simulink model "rc_node"  (Simulink 7.8)
settings: Solver=FixedStepDiscrete  SolverMode=SingleTasking  StartTime=0.0  StopTime=10.0  FixedStep=0.01  RelTol=1e-3
InitFcn:
  | clear all;
  | RcNodeInit
values from neighbouring files (symbols this model uses):
  MaxPwmIn = 0.0025    [RcNodeInit.m]
  T_step = 0.01    [RcNodeInit.m]
undefined symbols (not defined in the file or in its folder): Acs300SendThrottleCommand, ANmax, DataEEInitAndClear, DataStoreSaveParameters, DiscIntNeverNeededParam, Ecan1Init, IC1max, IC2max, IC7max, IC8max, Init_onlyOnce, Init_Reset, NodeTransmitStatus, RcNodeInit, RudderSendAngleCommand, RudderStartCalibration, TransmitStatus, u1, u2
libraries: simulink x35, dsPICdrivers x19, simulink_need_slupdate x1, ecan_dspic x1
(part 1 of 2)
CloseFcn:
  | rtwprivate ssgencode ModelCloseRequest rc_node
settings Model: Creator=bwmairs  LastModifiedBy=Bryant
settings OptimizationCC: BlockReduction=off  InlineParams=on  InlineInvariantSignals=on  PassReuseOutputArgsAs=Individual arguments  ZeroExternalMemoryAtStartup=off  ZeroInternalMemoryAtStartup=off  InitFltsAndDblsToZero=on  NoFixptDivByZeroProtection=on  EfficientFloat2IntCast=on  OptimizeModelRefInitCode=on
settings DebuggingCC: ReadBeforeWriteMsg=DisableAll  WriteAfterWriteMsg=DisableAll  WriteAfterReadMsg=DisableAll  UnderspecifiedInitializationDetection=Simplified  ParameterOverflowMsg=warning  FcnCallInpInsideContextMsg=Use local settings  UniqueDataStoreMsg=error
settings HardwareCC: ProdBitPerInt=16  ProdBitPerPointer=16  ProdIntDivRoundTo=Zero  ProdEndianess=LittleEndian  ProdWordSize=16  ProdHWDeviceType=16-bit Generic
settings ModelReferenceCC: ModelReferenceNumInstancesAllowed=Single
settings SFSimCC: SimParseCustomCode=off
settings RTWCC: SystemTargetFile=dspic.tlc  GenCodeOnly=on  MakeCommand=make_CreateMPLAB  TemplateMakefile=dspic_pic30_gcc.tmf  PostCodeGenCommand=dsPIC_Compile()  Description=Embedded Target for Microchip dsPIC (real-time)  ProcessScript=dspic_make_rtw_hook  CustomInclude=../Libs/C  RTWCompilerOptimization=On
settings RTWCC: CustomSource=|
  | ../Libs/C/Conversions.c
  | ../Libs/C/Nmea2000.c
  | ../Libs/C/Nmea2000Encode.c
  | ../Libs/C/Uart1.c
  | ../Libs/C/DEE.c
  | ../Libs/C/DEES.s
  | ../Libs/C/Traps.c
  | ../Libs/C/CanMessages.c
  | ../Libs/C/Acs300.c
  | ../Libs/C/Rudder.c
  | ../Libs/C/Node.c
  | ../Libs/C/CircularBuffer.c
  | ../Libs/C/Ecan1.c
  | ../Libs/C/Parameters.c
  | ../Libs/C/DataStore.c
  | 
  | clib/RcNode.c
  | clib/ParametersHelper.c
settings CodeAppCC: IgnoreCustomStorageClasses=off  IgnoreTestpoints=on
settings STFCustomTargetCC: TargetFunctionLibrary=C89/C90 (ANSI)  IncludeMdlTerminateFcn=off  GeneratePreprocessorConditionals=Use local settings  CombineOutputUpdateFcns=on  SuppressErrorStatus=on  ERTCustomFileBanners=on  SupportComplex=off  SupportContinuousTime=off  SupportNonInlinedSFcns=off  SystemTargetFile=dspic.tlc
settings ERTTargetCC: TargetFunctionLibrary=C89/C90 (ANSI)  MultiwordLength=2048  ParMdlRefBuildCompliant=off  CompOptLevelCompliant=off  ConcurrentExecutionCompliant=off  IncludeMdlTerminateFcn=off  SuppressErrorStatus=on  ERTFirstTimeCompliant=off  SupportComplex=off  ModelStepFunctionPrototypeControlCompliant=off  CPPClassGenCompliant=off  ExtModeMexFile=ext_serial_win32_comm  InlinedParameterPlacement=NonHierarchical  ERTSrcFileBannerTemplate=dsPIC_code_template.cgt  ERTHdrFileBannerTemplate=dsPIC_code_template.cgt  ERTDataSrcFileTemplate=dsPIC_code_template.cgt  ERTDataHdrFileTemplate=dsPIC_code_template.cgt  ERTCustomFileTemplate=dsPIC_main.tlc  SuppressUnreachableDefaultCases=off
settings CustomProperty: DataType=string  Value=C:\PROGRA~1\MATLAB\R2011b\bin\win64\gmake

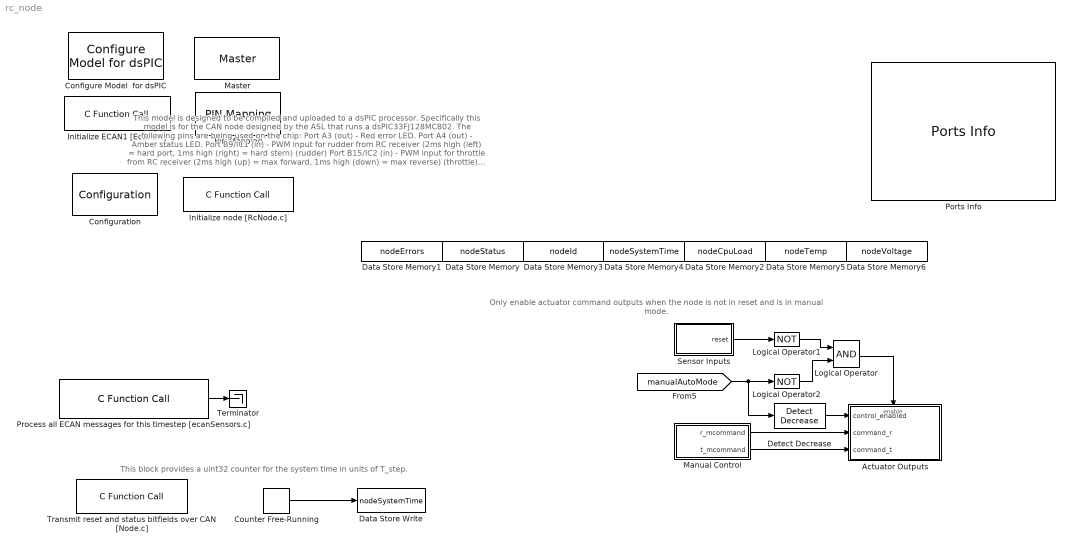
== system rc_node ==
  note: This model is designed to be compiled and uploaded to a dsPIC processor.
      | Specifically this model is for the CAN node designed by the ASL that runs a dsPIC33FJ128MC802.
      | The following pins are being used on the chip:
      | Port A3 (out) - Red error LED.
      | Port A4 (out) - Amber status LED.
      | Port B9/IC1 (in) - PWM input for rudder from RC receiver (2ms high (left) = hard port, 1ms high (right) = hard stern) (rudder)
      | Port B15/IC2 (in) - PWM input for throttle from RC receiver (2ms high (up) = max forward, 1ms high (down) = max reverse) (throttle)
      | Port B10/IC7 (in) - PWM input for control mode from RC receiver (2ms high (down) = manual control, 1ms high (up) = auto. control) (gear)
      | Ports B6/B7 (in/out) - Pins required for the ECAN1 peripheral. This is used for controlling the propeller motor.
      | Port B4/B5 (in/out) - UART1 transmission line.
      |
      | Switching between the autonomous controller and manual control involves using the landing gear channel. When
      | it's enabled, it's under autonomous control. This can only be changed when the RC transmitter is on and connected and
      | is never changed otherwise.
      |
      | Additionally a rudder calibration command can be sent by being in manual mode and toggling channel 5, the aileron channel, left-right-left.
      | To do it a second time you need to switch out of and back into manual mode.
  note: This block provides a uint32 counter for the system time in units of T_step.
  note: Only enable actuator command outputs when the node is not in
      | reset and is in manual mode.
  Actuator Outputs : Subsystem
  Configuration : dsPICdrivers/Configuration  double64=on
  Configure Model  for dsPIC : dsPICdrivers/Simulink Configuration/Configure Model  for dsPIC
  Counter Free-Running : simulink/Sources/Counter Free-Running  NumBits=32  tsamp=T_step
  Data Store Memory : DataStoreMemory  DataStoreName=nodeStatus  ReadBeforeWriteMsg=warning  WriteAfterWriteMsg=warning  WriteAfterReadMsg=warning  OutDataTypeStr=uint16
      settings: RTWStateStorageClass=ImportedExtern
  Data Store Memory1 : DataStoreMemory  DataStoreName=nodeErrors  ReadBeforeWriteMsg=warning  WriteAfterWriteMsg=warning  WriteAfterReadMsg=warning  OutDataTypeStr=uint16
      settings: RTWStateStorageClass=ImportedExtern
  Data Store Memory2 : DataStoreMemory  DataStoreName=nodeCpuLoad  ReadBeforeWriteMsg=warning  WriteAfterWriteMsg=warning  WriteAfterReadMsg=warning  OutDataTypeStr=uint8
      settings: RTWStateStorageClass=ImportedExtern
  Data Store Memory3 : DataStoreMemory  DataStoreName=nodeId  ReadBeforeWriteMsg=warning  WriteAfterWriteMsg=warning  WriteAfterReadMsg=warning  OutDataTypeStr=uint8
      settings: RTWStateStorageClass=ImportedExtern
  Data Store Memory4 : DataStoreMemory  DataStoreName=nodeSystemTime  ReadBeforeWriteMsg=warning  WriteAfterWriteMsg=warning  WriteAfterReadMsg=warning  OutDataTypeStr=uint32
      settings: RTWStateStorageClass=ImportedExtern
  Data Store Memory5 : DataStoreMemory  DataStoreName=nodeTemp  ReadBeforeWriteMsg=warning  WriteAfterWriteMsg=warning  WriteAfterReadMsg=warning  OutDataTypeStr=int8
      settings: RTWStateStorageClass=ImportedExtern
  Data Store Memory6 : DataStoreMemory  DataStoreName=nodeVoltage  ReadBeforeWriteMsg=warning  WriteAfterWriteMsg=warning  WriteAfterReadMsg=warning  OutDataTypeStr=uint8
      settings: RTWStateStorageClass=ImportedExtern
  Data Store Write : DataStoreWrite  DataStoreName=nodeSystemTime
  Detect Decrease : simulink/Logic and Bit Operations/Detect Decrease  vinit=0.0  InputProcessing=Inherited  OutDataTypeStr=uint8
  Initialize ECAN1 [Ecan1.c] : dsPICdrivers/OTHERS/C Function Call  Tag=dsPIC_dsPIC_CFunctionCall  FctUpdate=None  fctName=Ecan1Init  INPUT_SIZE=1  INPUT1=--  INPUT2=--  INPUT3=--  OUTPUT_SIZE=1  OUTPUT1=--  SampleTime=Inf  InputType=[]  OutputType=[]  FctDeclaration=extern void Ecan1Init();  FctCall=Ecan1Init();  OrderingInOutPopup=None  FctStart=Start Function (Call once and only once)  FctStart_Name=Ecan1Init  FctStart_Declaration=inline extern void Ecan1Init();  FctStart_Call=Ecan1Init();  FctInit=None  FctInit_Name=Init_Reset  FctInit_Declaration=inline extern void Init_Reset();  FctInit_Call=Init_Reset();  PinDigitalInput=[]  PinDigitalOutput=[]  AnalogueInput=[]
  Initialize node [RcNode.c] : dsPICdrivers/OTHERS/C Function Call  Tag=dsPIC_dsPIC_CFunctionCall  FctUpdate=None  fctName=TransmitStatus  INPUT_SIZE=1  INPUT1=--  INPUT2=--  INPUT3=--  OUTPUT_SIZE=1  OUTPUT1=--  SampleTime=-1  InputType=[]  OutputType=[]  FctDeclaration=extern void TransmitStatus();  FctCall=TransmitStatus();  OrderingInOutPopup=None  FctStart=Start Function (Call once and only once)  FctStart_Name=RcNodeInit  FctStart_Declaration=inline extern void RcNodeInit();  FctStart_Call=RcNodeInit();  FctInit=None  FctInit_Name=Init_Reset  FctInit_Declaration=inline extern void Init_Reset();  FctInit_Call=Init_Reset();  PinDigitalInput=[]  PinDigitalOutput=[]  AnalogueInput=[]
  Logical Operator : Logic  AllPortsSameDT=off  OutDataTypeStr=boolean
  Logical Operator1 : Logic  Operator=NOT  AllPortsSameDT=off  OutDataTypeStr=boolean
  Logical Operator2 : Logic  Operator=NOT  AllPortsSameDT=off  OutDataTypeStr=boolean
  Manual Control : Subsystem
  Master : dsPICdrivers/Master  Tag=dsPIC_MASTER  Priority=1  TimeStepType=Timer1  picType=33fj128MC802  fcy=40008571.4286  Quartz_33f=8e6  PLLActive_33f=on  fcyDesired_33f=40000000  tmr1="[8  50010  -0.00057131]"  tmr1Info="Time Step : 0.01  ;   Error : -0.00057131%  PR1=50010"  tmr2345="[8  0  0  0]"  tmr2345cfg=[-1 -1 -1 -1]  IOautoConf=on  typePort="[ 0   8   0  10  10   0   0   0   0   0   0   0   0   0   0   0   0   0   0   8  22   0   0  23   0  22  22   0   0   0  22  22   0   0   0   0   0   0   0   0   0   0   0   0   0   0   0   0   0   0   0   0   0   0   0   0   0   0   0   0   0   0   0   0   0   0   0   0   0   0   0   0   0   0   0   0   0   0   0   0   0   0   0   0   0   0   0   0   0   0   0   0   0   0   0   0   0   0   0   0   0   0   0   0   0   0   0   0   0   0   0   0 ]"  TRIS="[ 65511  65407  65535  65535  65535  65535  65535 ]"  ADPCFG=0  MasterBusyPort=None  MasterOverloadPort=None  FOSC=Internal Fast RC 7.37Mhz  ClockSwitchMonitor=Both disabled  TempProtection_33f=TEMP_ON  FPBOR=<empty>  PWRT=disable  MCLR=<empty>  ICD=ICS_PGD3  JTAGEN=JTAGEN_OFF  PowerSave=off  OverrideFcy=off  NewFcy=1e6  PR2345="[65535  65535  65535  65535]"
  PIN Mapping : dsPICdrivers/Peripheral MAPPING/PIN Mapping  Tag=dsPIC_PIN_Mapping  in_INT1=Not tied (VSS)  in_INT2=Not tied (VSS)  in_T2CK=Not tied (VSS)  in_T3CK=Not tied (VSS)  in_T4CK=Not tied (VSS)  in_T5CK=Not tied (VSS)  in_IC1=tied to RP9  in_IC2=tied to RP15  in_IC7=tied to RP10  in_IC8=tied to RP14  out_OC1=Not changed  out_OC2=Not changed  out_OC3=Not changed  out_OC4=Not changed  in_OCFA=Not tied (VSS)  in_FLTA1=Not tied (VSS)  in_FLTA2=Not tied (VSS)  in_QEA1=Not tied (VSS)  in_QEB1=Not tied (VSS)  in_INDX1=Not tied (VSS)  out_UPDN1=Not changed  out_UPDN2=Not changed  in_QEA2=Not tied (VSS)  in_QEB2=Not tied (VSS)  in_INDX2=Not tied (VSS)  in_U1RX=Not changed  out_U1TX=Not changed  in_U1CTS=Not tied (VSS)  out_U1RTS=Not changed  in_U2RX=Not changed  out_U2TX=Not changed  in_U2CTS=Not tied (VSS)  out_U2RTS=Not changed  in_SDI1=Not tied (VSS)  out_SDO1=Not changed  in_SCK1=Not tied (VSS)  out_SCK1OUT=Not changed  in_SS1=Not tied (VSS)  out_SS1OUT=Not changed  in_SDI2=Not tied (VSS)  out_SDO2=Not changed  in_SCK2=Not tied (VSS)  out_SCK2OUT=Not changed  in_SS2=Not tied (VSS)  out_SS2OUT=Not changed  in_C1RX=tied to RP4  out_C1TX=tied to RP7  out_C1OUT=Not changed  out_C2OUT=Not changed
  Ports Info : dsPICdrivers/Ports Info  Tag=dsPIC_PortInfo
  Process all ECAN messages for this timestep [ecanSensors.c] : dsPICdrivers/OTHERS/C Function Call  Tag=dsPIC_dsPIC_CFunctionCall  FctUpdate=Output Function  fctName=ProcessAllEcanMessages  INPUT_SIZE=1  INPUT1=--  INPUT2=--  INPUT3=--  OUTPUT_SIZE=1  OUTPUT1=uint8  SampleTime=T_step  InputType=[ ]  OutputType=[ 2 ]  FctDeclaration=extern uint8_T ProcessAllEcanMessages();  FctCall=%y1 = ProcessAllEcanMessages();  OrderingInOutPopup=None  FctStart=None  FctStart_Name=Init_onlyOnce  FctStart_Declaration=inline extern void Init_onlyOnce();  FctStart_Call=Init_onlyOnce();  FctInit=None  FctInit_Name=Init_Reset  FctInit_Declaration=inline extern void Init_Reset();  FctInit_Call=Init_Reset();  PinDigitalInput=[]  PinDigitalOutput=[]  AnalogueInput=[]
  Sensor Inputs : Subsystem
  Terminator : Terminator
  Transmit reset and status bitfields over CAN [Node.c] : dsPICdrivers/OTHERS/C Function Call  Tag=dsPIC_dsPIC_CFunctionCall  FctUpdate=Output Function  fctName=NodeTransmitStatus  INPUT_SIZE=1  INPUT1=--  INPUT2=--  INPUT3=--  OUTPUT_SIZE=1  OUTPUT1=--  SampleTime=0.5  InputType=[ ]  OutputType=[ ]  FctDeclaration=extern void NodeTransmitStatus();  FctCall=NodeTransmitStatus();  OrderingInOutPopup=None  FctStart=None  FctStart_Name=DataEEInitAndClear  FctStart_Declaration=inline extern void DataEEInitAndClear();  FctStart_Call=DataEEInitAndClear();  FctInit=None  FctInit_Name=Init_Reset  FctInit_Declaration=inline extern void Init_Reset();  FctInit_Call=Init_Reset();  PinDigitalInput=[]  PinDigitalOutput=[]  AnalogueInput=[]
  wires:
  Process all ECAN messages for this timestep [ecanSensors.c]/1 -> Terminator/1
  Sensor Inputs/1(reset) -> Logical Operator1/1
  Manual Control/1(r_mcommand) -> Actuator Outputs/2(command_r)
  Manual Control/2(t_mcommand) -> Actuator Outputs/3(command_t)
  Logical Operator1/1 -> Logical Operator/1
  Counter Free-Running/1 -> Data Store Write/1
  [manualAutoMode] -> Logical Operator2/1, Detect Decrease/1
  Logical Operator/1 -> Actuator Outputs/Enable
  Logical Operator2/1 -> Logical Operator/2
  Detect Decrease/1 -> Actuator Outputs/1(control_enabled)

== system rc_node/Actuator Outputs ==
  note: Propulsion is controlled here via a CAN interface to the motor driver board.
      | ECAN1 is used and several possible commands are transmitted: enable, disable,
      | or change speed, with speed being between -1023 and 1023 taken as a fraction
      | of total speed (1023).
  note: Rudder commands are controlled via a CAN interface to a CAN_node controller
      | at the stern of the vessel.
  note: Actuator messages are only transmit when the command signal has changed,
      | though when the device is switched over to manual control, messages are
      | transmit as well.
  control_enabled : Inport
  command_r : Inport  Port=2
  command_t : Inport  Port=3
  Enable : EnablePort
  Detect Change : simulink/Logic and Bit Operations/Detect Change  vinit=0  InputProcessing=Inherited  OutDataTypeStr=uint8
  Detect Change1 : simulink/Logic and Bit Operations/Detect Change  vinit=0  InputProcessing=Inherited  OutDataTypeStr=uint8
  Logical Operator : Logic  Operator=OR  AllPortsSameDT=off  OutDataTypeStr=boolean
  Logical Operator1 : Logic  Operator=OR  AllPortsSameDT=off  OutDataTypeStr=boolean
  Transmit Angle Command : Subsystem  TreatAsAtomicUnit=on
  Transmit Throttle Command : Subsystem  TreatAsAtomicUnit=on
  wires:
  command_r/1 -> Detect Change/1, Transmit Angle Command/1(r_angle)
  command_t/1 -> Transmit Throttle Command/1(t_cmd), Detect Change1/1
  Logical Operator/1 -> Transmit Angle Command/Trigger
  Detect Change/1 -> Logical Operator/2
  control_enabled/1 -> Logical Operator/1, Logical Operator1/1
  Logical Operator1/1 -> Transmit Throttle Command/Trigger
  Detect Change1/1 -> Logical Operator1/2

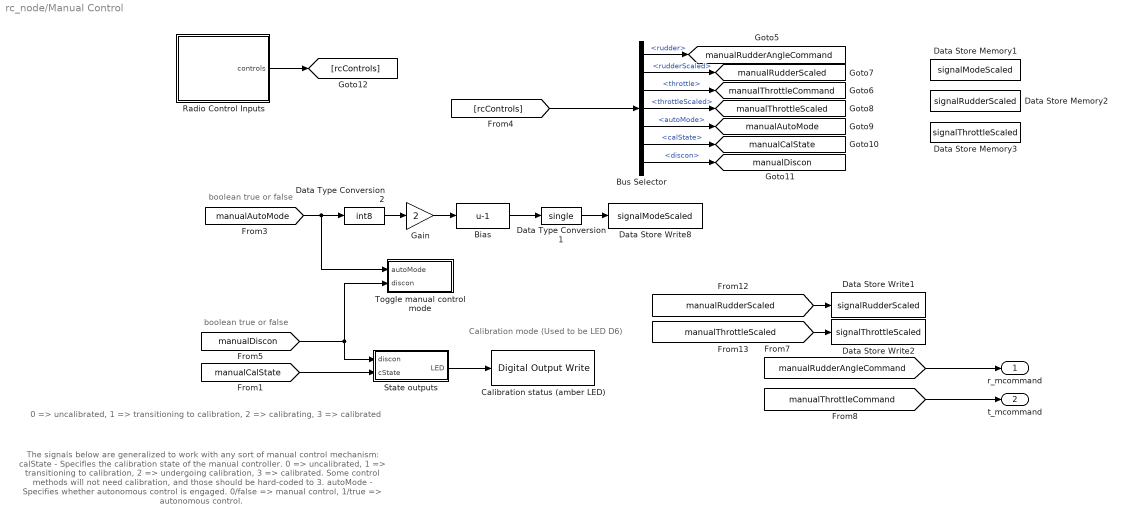
== system rc_node/Manual Control ==
  note: The signals below are generalized to work with any sort of manual control mechanism:
      | calState - Specifies the calibration state of the manual controller.
      |                 0 => uncalibrated, 1 => transitioning to calibration, 2 => undergoing calibration, 3 => calibrated. Some control methods will not need calibration, and those should be hard-coded to 3.
      | autoMode - Specifies whether autonomous control is engaged. 0/false => manual control, 1/true => autonomous control.
  note: boolean true or false
  note: boolean true or false
  note: 0 => uncalibrated,
      | 1 => transitioning to calibration,
      | 2 => calibrating,
      | 3 => calibrated
  note: Calibration mode
      | (Used to be LED D6)
  Bias : Bias  Bias=-1
  Bus Selector : BusSelector  OutputSignals=rudder,rudderScaled,throttle,throttleScaled,autoMode,calState,discon
  Calibration status (amber LED) : dsPICdrivers/Digital I//O/Digital Output Write  Tag=dsPIC_Digital_Output  Priority=5  PORT=A  Pin=[4]  Simultaneous=off  OrderingInOutPopup=None
  Data Store Memory1 : DataStoreMemory  DataStoreName=signalModeScaled  ReadBeforeWriteMsg=warning  WriteAfterWriteMsg=warning  WriteAfterReadMsg=warning  OutDataTypeStr=single
      settings: RTWStateStorageClass=ExportedGlobal
  Data Store Memory2 : DataStoreMemory  DataStoreName=signalRudderScaled  ReadBeforeWriteMsg=warning  WriteAfterWriteMsg=warning  WriteAfterReadMsg=warning  OutDataTypeStr=single
      settings: RTWStateStorageClass=ExportedGlobal
  Data Store Memory3 : DataStoreMemory  DataStoreName=signalThrottleScaled  ReadBeforeWriteMsg=warning  WriteAfterWriteMsg=warning  WriteAfterReadMsg=warning  OutDataTypeStr=single
      settings: RTWStateStorageClass=ExportedGlobal
  Data Store Write1 : DataStoreWrite  DataStoreName=signalRudderScaled
  Data Store Write2 : DataStoreWrite  DataStoreName=signalThrottleScaled
  Data Store Write8 : DataStoreWrite  DataStoreName=signalModeScaled  DataStoreElements=signalModeScaled
  Data Type Conversion1 : DataTypeConversion  OutDataTypeStr=single  RndMeth=Simplest
  Data Type Conversion2 : DataTypeConversion  OutDataTypeStr=int8  RndMeth=Simplest
  Gain : Gain  Gain=2  OutDataTypeStr=Inherit: Same as input  ParamDataTypeStr=Inherit: Same as input
  Radio Control Inputs : Subsystem
  State outputs : Subsystem
  Toggle manual control mode : Subsystem
  r_mcommand : Outport
  t_mcommand : Outport  Port=2
  tag scope: manualAutoMode=global, manualCalState=global, manualDiscon=global, manualRudderAngleCommand=global, manualRudderScaled=global, manualThrottleCommand=global, manualThrottleScaled=global
  wires:
  State outputs/1(LED) -> Calibration status (amber LED)/1
  Bias/1 -> Data Type Conversion1/1
  Gain/1 -> Bias/1
  Radio Control Inputs/1(controls) -> [rcControls]
  Bus Selector/1 -> [manualRudderAngleCommand]  "<rudder>"
  Bus Selector/3 -> [manualThrottleCommand]  "<throttle>"
  Bus Selector/2 -> [manualRudderScaled]  "<rudderScaled>"
  Bus Selector/4 -> [manualThrottleScaled]  "<throttleScaled>"
  Bus Selector/5 -> [manualAutoMode]  "<autoMode>"
  Bus Selector/6 -> [manualCalState]  "<calState>"
  Bus Selector/7 -> [manualDiscon]  "<discon>"
  [manualAutoMode] -> Data Type Conversion2/1, Toggle manual control mode/1(autoMode)
  [manualDiscon] -> State outputs/1(discon), Toggle manual control mode/2(discon)
  [manualCalState] -> State outputs/2(cState)
  [manualRudderAngleCommand] -> r_mcommand/1
  [manualThrottleCommand] -> t_mcommand/1
  [manualThrottleScaled] -> Data Store Write2/1
  [manualRudderScaled] -> Data Store Write1/1
  [rcControls] -> Bus Selector/1
  Data Type Conversion1/1 -> Data Store Write8/1
  Data Type Conversion2/1 -> Gain/1

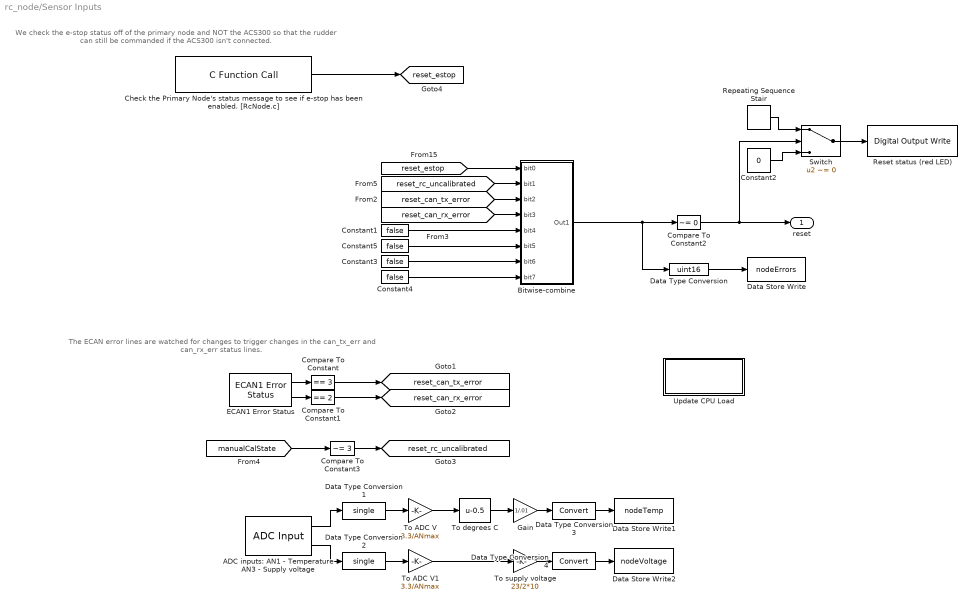
== system rc_node/Sensor Inputs ==
  note: The ECAN error lines are watched for changes to trigger changes
      | in the can_tx_err and can_rx_err status lines.
  note: We check the e-stop status off of the primary node and NOT the ACS300 so that
      | the rudder can still be commanded if the ACS300 isn't connected.
  ADC inputs: AN1 - Temperature AN3 - Supply voltage : dsPICdrivers/Peripheral I//O/ADC Input  Tag=dsPIC_ADC  Priority=5  ADC_TYPE=12 bits  ADC_MODE=Continuous sampling & get last channel value  NbrSampleStep=1  VoltRefpopup="AVdd  -  AVss"  OutFormatBitspopup=0000 dddd dddd dddd : Integer  InterruptPriority=6  ANCHANNELS=[1 5]  MaxName=ANmax = 4095  Rin=0  ADCS=53  SAMC=1  Temperature=25  DMAChannel=7  SampleTime=T_step  Status="OK  |  Tsmp=6.749e-007 |  T/Channel=1.012e-005 |  Tall=2.025e-005"  SSRC=auto convert
  Bitwise-combine : Subsystem
  Check the Primary Node's status message to see if e-stop has been enabled. [RcNode.c] : dsPICdrivers/OTHERS/C Function Call  Tag=dsPIC_dsPIC_CFunctionCall  FctUpdate=Output Function  fctName=GetEstopStatus  INPUT_SIZE=1  INPUT1=--  INPUT2=--  INPUT3=--  OUTPUT_SIZE=1  OUTPUT1=uint8  SampleTime=T_step  InputType=[ ]  OutputType=[ 2 ]  FctDeclaration=extern uint8_T GetEstopStatus();  FctCall=%y1 = GetEstopStatus();  OrderingInOutPopup=None  FctStart=None  FctStart_Name=Init_onlyOnce  FctStart_Declaration=inline extern void Init_onlyOnce();  FctStart_Call=Init_onlyOnce();  FctInit=None  FctInit_Name=Init_Reset  FctInit_Declaration=inline extern void Init_Reset();  FctInit_Call=Init_Reset();  PinDigitalInput=[]  PinDigitalOutput=[]  AnalogueInput=[]
  Compare To Constant : simulink/Logic and Bit Operations/Compare To Constant  relop===  const=3  OutDataTypeStr=boolean
  Compare To Constant1 : simulink/Logic and Bit Operations/Compare To Constant  relop===  const=2  OutDataTypeStr=boolean
  Compare To Constant2 : simulink/Logic and Bit Operations/Compare To Constant  relop=~=  const=0  OutDataTypeStr=boolean
  Compare To Constant3 : simulink/Logic and Bit Operations/Compare To Constant  relop=~=  const=3  OutDataTypeStr=boolean
  Constant{1,3..5} (4 alike) : Constant  Value=false  OutDataTypeStr=boolean
  Constant2 : Constant  Value=0  OutDataTypeStr=boolean
  Data Store Write : DataStoreWrite  DataStoreName=nodeErrors
  Data Store Write1 : DataStoreWrite  DataStoreName=nodeTemp
  Data Store Write2 : DataStoreWrite  DataStoreName=nodeVoltage
  Data Type Conversion : DataTypeConversion  OutDataTypeStr=uint16  RndMeth=Simplest
  Data Type Conversion1 : DataTypeConversion  OutDataTypeStr=single
  Data Type Conversion2 : DataTypeConversion  OutDataTypeStr=single
  Data Type Conversion3 : DataTypeConversion  RndMeth=Simplest
  Data Type Conversion4 : DataTypeConversion  RndMeth=Simplest
  ECAN1 Error Status : ecan_dspic/ECAN1 Error Status  ecan1_error_sample_time=T_step
  Gain : Gain  Gain=1/.01  RndMeth=Simplest
  Repeating Sequence Stair : simulink/Sources/Repeating Sequence Stair  OutValues=[1 0]  tsamp=.5  OutMin=[]  OutMax=[]  OutDataTypeStr=fixdt('boolean')  OutputDataTypeScalingMode=Specify via dialog  OutDataType=fixdt('boolean')  ConRadixGroup=Best Precision: Vector-wise  OutScaling=[]
  Reset status (red LED) : dsPICdrivers/Digital I//O/Digital Output Write  Tag=dsPIC_Digital_Output  Priority=5  PORT=A  Pin=[3]  Simultaneous=off  OrderingInOutPopup=None
  Switch : Switch  Criteria=u2 ~= 0
  To ADC V : Gain  Gain=3.3/ANmax
  To ADC V1 : Gain  Gain=3.3/ANmax
  To degrees C : Bias  Bias=-0.5
  To supply voltage : Gain  Gain=23/2*10  RndMeth=Simplest
  Update CPU Load : Subsystem
      mask Display: disp('');
  reset : Outport
  tag scope: reset_can_rx_error=global, reset_can_tx_error=global, reset_estop=global, reset_rc_uncalibrated=global
  wires:
  Check the Primary Node's status message to see if e-stop has been enabled. [RcNode.c]/1 -> [reset_estop]
  ECAN1 Error Status/1 -> Compare To Constant/1
  ECAN1 Error Status/2 -> Compare To Constant1/1
  Compare To Constant1/1 -> [reset_can_rx_error]
  Compare To Constant/1 -> [reset_can_tx_error]
  Constant2/1 -> Switch/3
  Repeating Sequence Stair/1 -> Switch/1
  Switch/1 -> Reset status (red LED)/1
  [reset_estop] -> Bitwise-combine/1(bit0)
  [reset_rc_uncalibrated] -> Bitwise-combine/2(bit1)
  [reset_can_tx_error] -> Bitwise-combine/3(bit2)
  [reset_can_rx_error] -> Bitwise-combine/4(bit3)
  Bitwise-combine/1(Out1) -> Compare To Constant2/1, Data Type Conversion/1
  Compare To Constant2/1 -> Switch/2, reset/1
  Constant3/1 -> Bitwise-combine/7(bit6)
  Constant4/1 -> Bitwise-combine/8(bit7)
  Data Type Conversion/1 -> Data Store Write/1
  Compare To Constant3/1 -> [reset_rc_uncalibrated]
  [manualCalState] -> Compare To Constant3/1
  Constant1/1 -> Bitwise-combine/5(bit4)
  Constant5/1 -> Bitwise-combine/6(bit5)
  To ADC V/1 -> To degrees C/1
  Data Type Conversion1/1 -> To ADC V/1
  ADC inputs: AN1 - Temperature AN3 - Supply voltage/1 -> Data Type Conversion1/1
  To degrees C/1 -> Gain/1
  Gain/1 -> Data Type Conversion3/1
  To ADC V1/1 -> To supply voltage/1
  Data Type Conversion2/1 -> To ADC V1/1
  To supply voltage/1 -> Data Type Conversion4/1
  ADC inputs: AN1 - Temperature AN3 - Supply voltage/2 -> Data Type Conversion2/1
  Data Type Conversion3/1 -> Data Store Write1/1
  Data Type Conversion4/1 -> Data Store Write2/1

== system rc_node/Actuator Outputs/Transmit Angle Command ==
  r_angle : Inport
  Trigger : TriggerPort
  Data Store Read1 : DataStoreRead  DataStoreName=nodeId
  Transmit rudder angle command [Rudder.c] : dsPICdrivers/OTHERS/C Function Call  Tag=dsPIC_dsPIC_CFunctionCall  FctUpdate=Output Function  fctName=RudderSendAngleCommand  INPUT_SIZE=1  INPUT1=uint8  INPUT2=real32  INPUT3=--  OUTPUT_SIZE=1  OUTPUT1=--  SampleTime=-1  InputType=[ 2 7 ]  OutputType=[ ]  FctDeclaration=extern void RudderSendAngleCommand(uint8_T u1, real32_T u2);  FctCall=RudderSendAngleCommand(%u1, %u2);  OrderingInOutPopup=None  FctStart=None  FctStart_Name=Init_onlyOnce  FctStart_Declaration=inline extern void Init_onlyOnce();  FctStart_Call=Init_onlyOnce();  FctInit=None  FctInit_Name=Init_Reset  FctInit_Declaration=inline extern void Init_Reset();  FctInit_Call=Init_Reset();  PinDigitalInput=[]  PinDigitalOutput=[]  AnalogueInput=[]
  wires:
  r_angle/1 -> Transmit rudder angle command [Rudder.c]/2
  Data Store Read1/1 -> Transmit rudder angle command [Rudder.c]/1

== system rc_node/Actuator Outputs/Transmit Throttle Command ==
  t_cmd : Inport
  Trigger : TriggerPort
  Transmit throttle angle command [Acs300.c] : dsPICdrivers/OTHERS/C Function Call  Tag=dsPIC_dsPIC_CFunctionCall  FctUpdate=Output Function  fctName=Acs300SendThrottleCommand  INPUT_SIZE=1  INPUT1=int16  INPUT2=--  INPUT3=--  OUTPUT_SIZE=1  OUTPUT1=--  SampleTime=-1  InputType=[ 3 ]  OutputType=[ ]  FctDeclaration=extern void Acs300SendThrottleCommand(int16_T u1);  FctCall=Acs300SendThrottleCommand(%u1);  OrderingInOutPopup=None  FctStart=None  FctStart_Name=Init_onlyOnce  FctStart_Declaration=inline extern void Init_onlyOnce();  FctStart_Call=Init_onlyOnce();  FctInit=None  FctInit_Name=Init_Reset  FctInit_Declaration=inline extern void Init_Reset();  FctInit_Call=Init_Reset();  PinDigitalInput=[]  PinDigitalOutput=[]  AnalogueInput=[]
  wires:
  t_cmd/1 -> Transmit throttle angle command [Acs300.c]/1

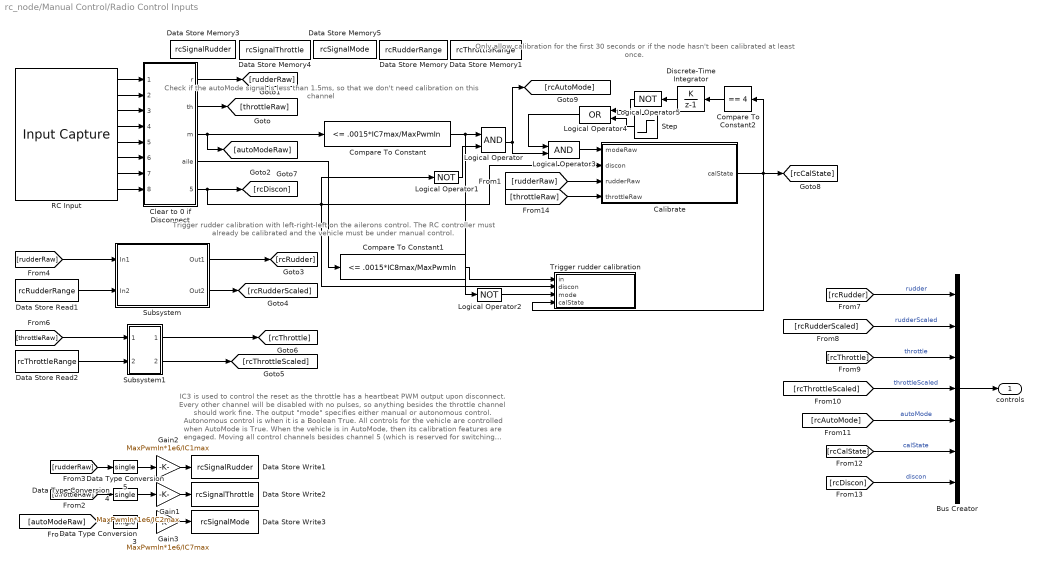
== system rc_node/Manual Control/Radio Control Inputs ==
  note: IC3 is used to control the reset as the throttle has a heartbeat PWM output upon disconnect.
      | Every other channel will be disabled with no pulses, so anything besides the throttle channel
      | should work fine.
      |
      | The output "mode" specifies either manual or autonomous control. Autonomous control is when
      | it is a Boolean True.
      |
      | All controls for the vehicle are controlled when AutoMode is True. When the vehicle is in
      | AutoMode, then its calibration features are engaged. Moving all control channels besides channel
      | 5 (which is reserved for switching AutoMode) will calibrate the controller to the proper values.
      |
      | As the vehicle enters reset automatically on startup, the proper way to calibrate the RC receiver is to
      | startup the vehicle, trigger RC calibration moving all of the control sticks excluding ch. 5 (landing gear),
      | and then switch the landing gear channel again and possibly once more to get into the manual control
      | mode.
      |
      | The output for rudder and throttle are all in the range -1..1000. -1 means disconnected,
      | while 0 is a low RC signal and 1000 is a high. These ranges also have deadbands: 4% at the low-end or
      | 8% around the center. This helps to keep the actuator dead if the user desires it.
  note: Check if the autoMode signal is less than 1.5ms,
      | so that we don't need calibration on this channel
  note: Only allow calibration for the first 30 seconds or if
      | the node hasn't been calibrated at least once.
  note: Trigger rudder calibration with left-right-left on the ailerons control. The RC controller must already be calibrated
      | and the vehicle must be under manual control.
  Bus Creator : BusCreator  Inputs=7
  Calibrate : Subsystem
  Clear to 0 if Disconnect : Subsystem
  Compare To Constant : simulink/Logic and Bit Operations/Compare To Constant  relop=<=  const=.0015*IC7max/MaxPwmIn  OutDataTypeStr=boolean
  Compare To Constant1 : simulink/Logic and Bit Operations/Compare To Constant  relop=<=  const=.0015*IC8max/MaxPwmIn  OutDataTypeStr=boolean
  Compare To Constant2 : simulink/Logic and Bit Operations/Compare To Constant  relop===  const=4  OutDataTypeStr=uint8
  Data Store Memory : DataStoreMemory  DataStoreName=rcRudderRange  ReadBeforeWriteMsg=warning  WriteAfterWriteMsg=warning  WriteAfterReadMsg=warning  InitialValue=[0 0]  OutDataTypeStr=uint16
      settings: RTWStateStorageClass=ImportedExtern
  Data Store Memory1 : DataStoreMemory  DataStoreName=rcThrottleRange  ReadBeforeWriteMsg=warning  WriteAfterWriteMsg=warning  WriteAfterReadMsg=warning  InitialValue=[8000 8000]  OutDataTypeStr=uint16
      settings: RTWStateStorageClass=ImportedExtern
  Data Store Memory3 : DataStoreMemory  DataStoreName=rcSignalRudder  ReadBeforeWriteMsg=warning  WriteAfterWriteMsg=warning  WriteAfterReadMsg=warning  OutDataTypeStr=uint16
      settings: RTWStateStorageClass=ExportedGlobal
  Data Store Memory4 : DataStoreMemory  DataStoreName=rcSignalThrottle  ReadBeforeWriteMsg=warning  WriteAfterWriteMsg=warning  WriteAfterReadMsg=warning  OutDataTypeStr=uint16
      settings: RTWStateStorageClass=ExportedGlobal
  Data Store Memory5 : DataStoreMemory  DataStoreName=rcSignalMode  ReadBeforeWriteMsg=warning  WriteAfterWriteMsg=warning  WriteAfterReadMsg=warning  OutDataTypeStr=uint16
      settings: RTWStateStorageClass=ExportedGlobal
  Data Store Read1 : DataStoreRead  DataStoreName=rcRudderRange  SampleTime=T_step
  Data Store Read2 : DataStoreRead  DataStoreName=rcThrottleRange  SampleTime=T_step
  Data Store Write1 : DataStoreWrite  DataStoreName=rcSignalRudder
  Data Store Write2 : DataStoreWrite  DataStoreName=rcSignalThrottle
  Data Store Write3 : DataStoreWrite  DataStoreName=rcSignalMode
  Data Type Conversion3 : DataTypeConversion  OutDataTypeStr=single  RndMeth=Simplest
  Data Type Conversion4 : DataTypeConversion  OutDataTypeStr=single  RndMeth=Simplest
  Data Type Conversion5 : DataTypeConversion  OutDataTypeStr=single  RndMeth=Simplest
  Discrete-Time Integrator : DiscreteIntegrator  IntegratorMethod=Accumulation: Forward Euler  SampleTime=T_step  LimitOutput=on  UpperSaturationLimit=1  ICPrevOutput=DiscIntNeverNeededParam  ICPrevScaledInput=DiscIntNeverNeededParam
  Gain1 : Gain  Gain=MaxPwmIn*1e6/IC2max  OutDataTypeStr=uint16  RndMeth=Simplest  ParamDataTypeStr=Inherit: Same as input
  Gain2 : Gain  Gain=MaxPwmIn*1e6/IC1max  OutDataTypeStr=uint16  RndMeth=Simplest  ParamDataTypeStr=Inherit: Same as input
  Gain3 : Gain  Gain=MaxPwmIn*1e6/IC7max  OutDataTypeStr=uint16  RndMeth=Simplest  ParamDataTypeStr=Inherit: Same as input
  Logical Operator : Logic  AllPortsSameDT=off  OutDataTypeStr=boolean
  Logical Operator1 : Logic  Operator=NOT  AllPortsSameDT=off  OutDataTypeStr=boolean
  Logical Operator2 : Logic  Operator=NOT  AllPortsSameDT=off  OutDataTypeStr=boolean
  Logical Operator3 : Logic  AllPortsSameDT=off  OutDataTypeStr=boolean
  Logical Operator4 : Logic  Operator=OR  AllPortsSameDT=off  OutDataTypeStr=boolean
  Logical Operator5 : Logic  Operator=NOT  AllPortsSameDT=off  OutDataTypeStr=boolean
  RC Input : dsPICdrivers/Peripheral I//O/Input Capture  Tag=dsPIC_PWM_IC  Priority=5  IntPriority=7  Channel=[1 2 7 8]  Channel_UP_Down_Periode="[1  1  1  1]"  MaxChannel="[0.0025      0.0025      0.0025      0.0025]"  SafeMarge="[1  1  1  1]"  MaxName=' IC1max , IC2max , IC7max , IC8max '  Precision="[13.6098      13.6098      13.6098      13.6098]"  Timer="[2  2  2  2]"  ChangeDetected="[2  2  2  2]"  ChangeDetectedPortRef=3  SampleTime=T_step  Status=Channel not available on selected target
  Step : Step  Time=30  Before=1  After=0  SampleTime=T_step
  Subsystem : Subsystem
  Subsystem1 : Subsystem
  Trigger rudder calibration : Subsystem  TreatAsAtomicUnit=on
  controls : Outport
  wires:
  Clear to 0 if Disconnect/3(m) -> [autoModeRaw], Compare To Constant/1
  Clear to 0 if Disconnect/2(th) -> [throttleRaw]
  Data Store Read2/1 -> Subsystem1/2(In2)
  Data Store Read1/1 -> Subsystem/2(In2)
  Subsystem1/1(Out1) -> [rcThrottle]
  RC Input/1 -> Clear to 0 if Disconnect/1(rudder_up)
  RC Input/2 -> Clear to 0 if Disconnect/2(rudder_fall)
  RC Input/3 -> Clear to 0 if Disconnect/3(throttle_up)
  RC Input/4 -> Clear to 0 if Disconnect/4(throttle_fall)
  Subsystem/1(Out1) -> [rcRudder]
  [rudderRaw] -> Subsystem/1(In1)
  Subsystem/2(Out2) -> [rcRudderScaled]
  [throttleRaw] -> Subsystem1/1(In1)
  Subsystem1/2(Out2) -> [rcThrottleScaled]
  Clear to 0 if Disconnect/5(discon) -> [rcDiscon], Logical Operator1/1, Calibrate/2(discon), Trigger rudder calibration/2(discon)
  [rudderRaw] -> Data Type Conversion5/1
  [throttleRaw] -> Data Type Conversion4/1
  Gain1/1 -> Data Store Write2/1
  Data Type Conversion4/1 -> Gain1/1
  Gain2/1 -> Data Store Write1/1
  Data Type Conversion5/1 -> Gain2/1
  Clear to 0 if Disconnect/1(r) -> [rudderRaw]
  Gain3/1 -> Data Store Write3/1
  Data Type Conversion3/1 -> Gain3/1
  [autoModeRaw] -> Data Type Conversion3/1
  Bus Creator/1 -> controls/1
  [rcDiscon] -> Bus Creator/7  "discon"
  [rcRudder] -> Bus Creator/1  "rudder"
  [rcRudderScaled] -> Bus Creator/2  "rudderScaled"
  [rcThrottle] -> Bus Creator/3  "throttle"
  [rcThrottleScaled] -> Bus Creator/4  "throttleScaled"
  [rcAutoMode] -> Bus Creator/5  "autoMode"
  [rcCalState] -> Bus Creator/6  "calState"
  Calibrate/1(calState) -> [rcCalState], Trigger rudder calibration/4(calState), Compare To Constant2/1
  Compare To Constant/1 -> Logical Operator/1, Logical Operator2/1
  Logical Operator/1 -> [rcAutoMode], Logical Operator3/2
  Logical Operator1/1 -> Logical Operator/2
  [rudderRaw] -> Calibrate/3(rudderRaw)
  [throttleRaw] -> Calibrate/4(throttleRaw)
  RC Input/5 -> Clear to 0 if Disconnect/5(mode_up)
  RC Input/6 -> Clear to 0 if Disconnect/6(mode_fall)
  Clear to 0 if Disconnect/4(aile) -> Compare To Constant1/1
  Compare To Constant1/1 -> Trigger rudder calibration/1(in)
  RC Input/8 -> Clear to 0 if Disconnect/8(ailerons_fall)
  RC Input/7 -> Clear to 0 if Disconnect/7(aile_up)
  Logical Operator2/1 -> Trigger rudder calibration/3(mode)
  Logical Operator3/1 -> Calibrate/1(modeRaw)
  Logical Operator4/1 -> Logical Operator3/1
  Discrete-Time Integrator/1 -> Logical Operator5/1
  Step/1 -> Logical Operator4/2
  Logical Operator5/1 -> Logical Operator4/1
  Compare To Constant2/1 -> Discrete-Time Integrator/1

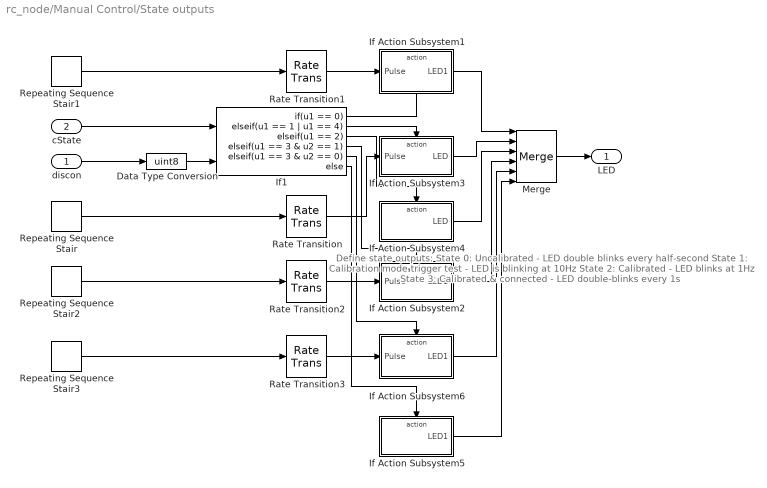
== system rc_node/Manual Control/State outputs ==
  note: Define state outputs:
      | State 0: Uncalibrated
      |   - LED double blinks every half-second
      | State 1: Calibration mode trigger test
      |   - LED is blinking at 10Hz
      | State 2: Calibrated
      |   - LED blinks at 1Hz
      | State 3: Calibrated & connected
      |   - LED double-blinks every 1s
  discon : Inport
  cState : Inport  Port=2
  Data Type Conversion : DataTypeConversion  OutDataTypeStr=uint8  RndMeth=Simplest
  If Action Subsystem1 : Subsystem  TreatAsAtomicUnit=on
  If Action Subsystem2 : Subsystem  TreatAsAtomicUnit=on
  If Action Subsystem3 : Subsystem  TreatAsAtomicUnit=on
  If Action Subsystem4 : Subsystem  TreatAsAtomicUnit=on
  If Action Subsystem5 : Subsystem  TreatAsAtomicUnit=on
  If Action Subsystem6 : Subsystem  TreatAsAtomicUnit=on
  If1 : If  NumInputs=2  IfExpression=u1 == 0  ElseIfExpressions=u1 == 1 | u1 == 4, u1 == 2, u1 == 3 & u2 == 1, u1 == 3 & u2 == 0
  Merge : Merge  Inputs=6  InitialOutput=false
  Rate Transition{,1..3} (4 alike) : RateTransition
  Repeating Sequence Stair : simulink/Sources/Repeating Sequence Stair  OutValues=[1 0]  tsamp=.1  OutMin=[]  OutMax=[]  OutDataTypeStr=fixdt('boolean')  OutputDataTypeScalingMode=Specify via dialog  OutDataType=fixdt('boolean')  ConRadixGroup=Best Precision: Vector-wise  OutScaling=[]
  Repeating Sequence Stair1 : simulink/Sources/Repeating Sequence Stair  OutValues=[1 0]  tsamp=.05  OutMin=[]  OutMax=[]  OutDataTypeStr=fixdt('boolean')  OutputDataTypeScalingMode=Specify via dialog  OutDataType=fixdt('boolean')  ConRadixGroup=Best Precision: Vector-wise  OutScaling=[]
  Repeating Sequence Stair2 : simulink/Sources/Repeating Sequence Stair  OutValues=[1 0]  tsamp=1  OutMin=[]  OutMax=[]  OutDataTypeStr=fixdt('boolean')  OutputDataTypeScalingMode=Specify via dialog  OutDataType=fixdt('boolean')  ConRadixGroup=Best Precision: Vector-wise  OutScaling=[]
  Repeating Sequence Stair3 : simulink/Sources/Repeating Sequence Stair  OutValues=[1 0 1 0 0 0 0 0 0 0]  tsamp=.1  OutMin=[]  OutMax=[]  OutDataTypeStr=fixdt('boolean')  OutputDataTypeScalingMode=Specify via dialog  OutDataType=fixdt('boolean')  ConRadixGroup=Best Precision: Vector-wise  OutScaling=[]
  LED : Outport
  wires:
  Rate Transition/1 -> If Action Subsystem3/1(Pulse)
  Repeating Sequence Stair/1 -> Rate Transition/1
  If Action Subsystem2/1(LED1) -> Merge/4
  If Action Subsystem4/1(LED) -> Merge/3
  If1/3 -> If Action Subsystem4/Action
  If1/4 -> If Action Subsystem2/Action
  If Action Subsystem3/1(LED) -> Merge/2
  If Action Subsystem1/1(LED1) -> Merge/1
  If1/2 -> If Action Subsystem3/Action
  If1/1 -> If Action Subsystem1/Action
  Merge/1 -> LED/1
  cState/1 -> If1/1
  Rate Transition1/1 -> If Action Subsystem1/1(Pulse)
  Repeating Sequence Stair1/1 -> Rate Transition1/1
  Rate Transition2/1 -> If Action Subsystem2/1(Pulse)
  Repeating Sequence Stair2/1 -> Rate Transition2/1
  If1/6 -> If Action Subsystem5/Action
  If Action Subsystem5/1(LED1) -> Merge/6
  Rate Transition3/1 -> If Action Subsystem6/1(Pulse)
  Repeating Sequence Stair3/1 -> Rate Transition3/1
  If Action Subsystem6/1(LED1) -> Merge/5
  If1/5 -> If Action Subsystem6/Action
  discon/1 -> Data Type Conversion/1
  Data Type Conversion/1 -> If1/2

== system rc_node/Manual Control/Toggle manual control mode ==
  note: This block implements event checking on the manual control and disconnected lines.
      | Whenever it changes this will update the system status accordingly.
  autoMode : Inport
  discon : Inport  Port=2
  Detect Change : simulink/Logic and Bit Operations/Detect Change  vinit=0  InputProcessing=Inherited  OutDataTypeStr=boolean
  Detect Change1 : simulink/Logic and Bit Operations/Detect Change  vinit=0  InputProcessing=Inherited  OutDataTypeStr=boolean
  If : If  NumInputs=4  IfExpression=(u1 | u3) & (u2 | u4)  ElseIfExpressions=(u1 | u3) & (~u2 & ~u4)  ShowElse=off
  If1 : If  NumInputs=2  IfExpression=u1 & u2  ElseIfExpressions=u1 & ~u2  ShowElse=off
  "RC transmitter is connected and the manual switch is engaged, so manual control is enabled." : Subsystem  TreatAsAtomicUnit=on
  "RC transmitter is connected, so update the status field" : Subsystem  TreatAsAtomicUnit=on
  "RC transmitter is disconnected, so update the status field" : Subsystem  TreatAsAtomicUnit=on
  "RC transmitter is disconnected, therefore manual control is disabled." : Subsystem  TreatAsAtomicUnit=on
  wires:
  autoMode/1 -> If/2, Detect Change/1
  If/1 -> "RC transmitter is disconnected, therefore manual control is disabled."/Action
  Detect Change/1 -> If/1
  If/2 -> "RC transmitter is connected and the manual switch is engaged, so manual control is enabled."/Action
  Detect Change1/1 -> If1/1, If/3
  discon/1 -> Detect Change1/1, If1/2, If/4
  If1/1 -> "RC transmitter is disconnected, so update the status field"/Action
  If1/2 -> "RC transmitter is connected, so update the status field"/Action

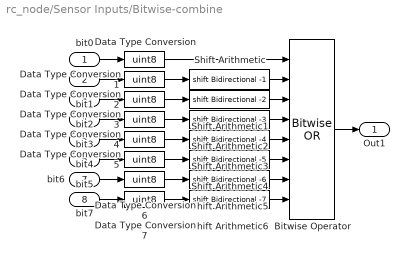
== system rc_node/Sensor Inputs/Bitwise-combine ==
  bit0 : Inport
  bit1 : Inport  Port=2
  bit2 : Inport  Port=3
  bit3 : Inport  Port=4
  bit4 : Inport  Port=5
  bit5 : Inport  Port=6
  bit6 : Inport  Port=7
  bit7 : Inport  Port=8
  Bitwise Operator : simulink/Logic and Bit Operations/Bitwise Operator  logicop=OR  UseBitMask=off  NumInputPorts=8  BitMask=bin2dec('11011001')  BitMaskRealWorld=Stored Integer
  Data Type Conversion{,1..7} (8 alike) : DataTypeConversion  OutDataTypeStr=uint8
  Shift Arithmetic : ArithShift  BitShiftNumber=-1
  Shift Arithmetic1 : ArithShift  BitShiftNumber=-2
  Shift Arithmetic2 : ArithShift  BitShiftNumber=-3
  Shift Arithmetic3 : ArithShift  BitShiftNumber=-4
  Shift Arithmetic4 : ArithShift  BitShiftNumber=-5
  Shift Arithmetic5 : ArithShift  BitShiftNumber=-6
  Shift Arithmetic6 : ArithShift  BitShiftNumber=-7
  Out1 : Outport
  wires:
  Shift Arithmetic/1 -> Bitwise Operator/2
  Shift Arithmetic1/1 -> Bitwise Operator/3
  Shift Arithmetic2/1 -> Bitwise Operator/4
  Data Type Conversion/1 -> Bitwise Operator/1
  Data Type Conversion1/1 -> Shift Arithmetic/1
  Data Type Conversion2/1 -> Shift Arithmetic1/1
  Data Type Conversion3/1 -> Shift Arithmetic2/1
  Data Type Conversion4/1 -> Shift Arithmetic3/1
  Shift Arithmetic3/1 -> Bitwise Operator/5
  Data Type Conversion5/1 -> Shift Arithmetic4/1
  Data Type Conversion6/1 -> Shift Arithmetic5/1
  Shift Arithmetic4/1 -> Bitwise Operator/6
  Shift Arithmetic5/1 -> Bitwise Operator/7
  Data Type Conversion7/1 -> Shift Arithmetic6/1
  Shift Arithmetic6/1 -> Bitwise Operator/8
  bit0/1 -> Data Type Conversion/1
  bit1/1 -> Data Type Conversion1/1
  bit2/1 -> Data Type Conversion2/1
  bit3/1 -> Data Type Conversion3/1
  Bitwise Operator/1 -> Out1/1
  bit4/1 -> Data Type Conversion4/1
  bit5/1 -> Data Type Conversion5/1
  bit6/1 -> Data Type Conversion6/1
  bit7/1 -> Data Type Conversion7/1

== system rc_node/Sensor Inputs/Update CPU Load ==
  Calculus Time Step : dsPICdrivers/OTHERS/Calculus Time Step  Tag=dsPIC_CalculusTimeStep  SampleTime=1  PR1chk=on
  Compare To Zero : simulink/Logic and Bit Operations/Compare To Zero  relop=~=  OutDataTypeStr=uint8
  Constant : Constant
  Data Store Write : DataStoreWrite  DataStoreName=nodeCpuLoad
  Data Type Conversion6 : DataTypeConversion  OutDataTypeStr=single
  Data Type Conversion7 : DataTypeConversion  OutDataTypeStr=single
  Gain : Gain  Gain=100  OutDataTypeStr=uint8
  Product : Product  Inputs=*/  RndMeth=Zero
  Switch : Switch  Criteria=u2 ~= 0
  wires:
  Calculus Time Step/1 -> Data Type Conversion6/1
  Calculus Time Step/2 -> Data Type Conversion7/1
  Product/1 -> Gain/1
  Gain/1 -> Data Store Write/1
  Data Type Conversion6/1 -> Product/1
  Data Type Conversion7/1 -> Switch/1, Compare To Zero/1
  Switch/1 -> Product/2
  Compare To Zero/1 -> Switch/2
  Constant/1 -> Switch/3

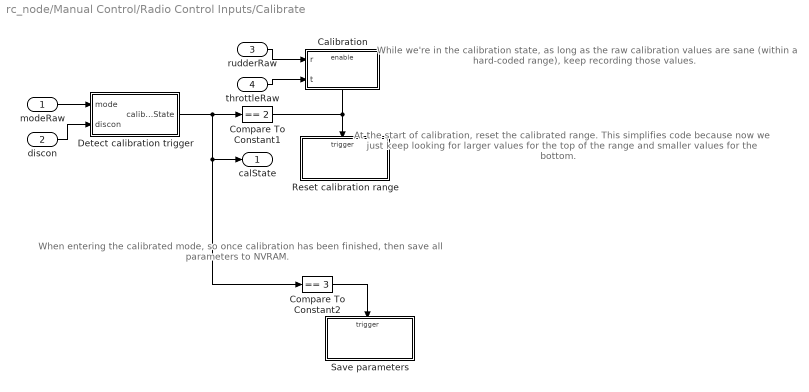
== system rc_node/Manual Control/Radio Control Inputs/Calibrate ==
  note: When entering the calibrated mode, so once calibration has been finished,
      | then save all parameters to NVRAM.
  note: While we're in the calibration state, as long as the raw calibration values are sane
      | (within a hard-coded range), keep recording those values.
  note: At the start of calibration, reset the calibrated range. This simplifies
      | code because now we just keep looking for larger values for the top
      | of the range and smaller values for the bottom.
  modeRaw : Inport
  discon : Inport  Port=2
  rudderRaw : Inport  Port=3
  throttleRaw : Inport  Port=4
  Calibration : Subsystem  TreatAsAtomicUnit=on
  Compare To Constant1 : simulink/Logic and Bit Operations/Compare To Constant  relop===  const=2  OutDataTypeStr=boolean
  Compare To Constant2 : simulink/Logic and Bit Operations/Compare To Constant  relop===  const=3  OutDataTypeStr=boolean
  Detect calibration trigger : Subsystem
  Reset calibration range : Subsystem  TreatAsAtomicUnit=on
  Save parameters : Subsystem  TreatAsAtomicUnit=on
  calState : Outport  SourceOfInitialOutputValue=Input signal
  wires:
  Detect calibration trigger/1(calibrateState) -> Compare To Constant1/1, calState/1, Compare To Constant2/1
  rudderRaw/1 -> Calibration/1(r)
  throttleRaw/1 -> Calibration/2(t)
  Compare To Constant1/1 -> Reset calibration range/Trigger, Calibration/Enable
  modeRaw/1 -> Detect calibration trigger/1(mode)
  discon/1 -> Detect calibration trigger/2(discon)
  Compare To Constant2/1 -> Save parameters/Trigger

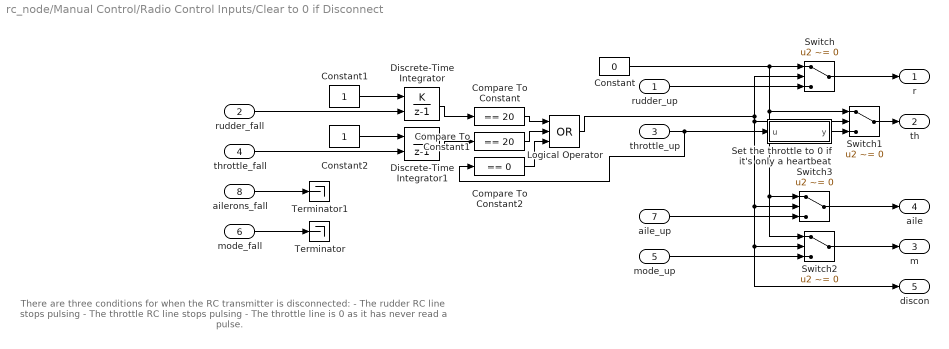
== system rc_node/Manual Control/Radio Control Inputs/Clear to 0 if Disconnect ==
  note: There are three conditions for when the RC transmitter is disconnected:
      |  - The rudder RC line stops pulsing
      |  - The throttle RC line stops pulsing
      |  - The throttle line is 0 as it has never read a pulse.
  rudder_up : Inport
  rudder_fall : Inport  Port=2
  throttle_up : Inport  Port=3
  throttle_fall : Inport  Port=4
  mode_up : Inport  Port=5
  mode_fall : Inport  Port=6
  aile_up : Inport  Port=7
  ailerons_fall : Inport  Port=8
  Compare To Constant : simulink/Logic and Bit Operations/Compare To Constant  relop===  const=20  OutDataTypeStr=boolean
  Compare To Constant1 : simulink/Logic and Bit Operations/Compare To Constant  relop===  const=20  OutDataTypeStr=boolean
  Compare To Constant2 : simulink/Logic and Bit Operations/Compare To Constant  relop===  const=0  OutDataTypeStr=boolean
  Constant : Constant  Value=0  OutDataTypeStr=int16
  Constant1 : Constant  OutDataTypeStr=uint8
  Constant2 : Constant  OutDataTypeStr=uint8
  Discrete-Time Integrator : DiscreteIntegrator  IntegratorMethod=Accumulation: Forward Euler  ExternalReset=level  SampleTime=-1  LimitOutput=on  UpperSaturationLimit=20  LowerSaturationLimit=0  ICPrevOutput=DiscIntNeverNeededParam  ICPrevScaledInput=DiscIntNeverNeededParam
  Discrete-Time Integrator1 : DiscreteIntegrator  IntegratorMethod=Accumulation: Forward Euler  ExternalReset=level  SampleTime=-1  LimitOutput=on  UpperSaturationLimit=20  LowerSaturationLimit=0  ICPrevOutput=DiscIntNeverNeededParam  ICPrevScaledInput=DiscIntNeverNeededParam
  Logical Operator : Logic  Operator=OR  Inputs=3  AllPortsSameDT=off  OutDataTypeStr=boolean
  Set the throttle to 0 if it's only a heartbeat : MATLAB Function  TreatAsAtomicUnit=on
  Switch{,1..3} (4 alike) : Switch  Criteria=u2 ~= 0  Threshold=40
  Terminator : Terminator
  Terminator1 : Terminator
  r : Outport
  th : Outport  Port=2
  m : Outport  Port=3
  aile : Outport  Port=4
  discon : Outport  Port=5
  wires:
  Switch1/1 -> th/1
  throttle_up/1 -> Compare To Constant2/1, Set the throttle to 0 if it's only a heartbeat/1(u)
  Switch/1 -> r/1
  rudder_up/1 -> Switch/3
  Constant/1 -> Switch/1, Switch1/1, Switch2/1, Switch3/1
  Switch2/1 -> m/1
  mode_up/1 -> Switch2/3
  rudder_fall/1 -> Discrete-Time Integrator/2
  Constant1/1 -> Discrete-Time Integrator/1
  throttle_fall/1 -> Discrete-Time Integrator1/2
  Constant2/1 -> Discrete-Time Integrator1/1
  Logical Operator/1 -> Switch/2, Switch1/2, Switch2/2, discon/1, Switch3/2
  Discrete-Time Integrator1/1 -> Compare To Constant1/1
  Discrete-Time Integrator/1 -> Compare To Constant/1
  Compare To Constant/1 -> Logical Operator/1
  Compare To Constant1/1 -> Logical Operator/2
  Compare To Constant2/1 -> Logical Operator/3
  Set the throttle to 0 if it's only a heartbeat/1(y) -> Switch1/3
  mode_fall/1 -> Terminator/1
  ailerons_fall/1 -> Terminator1/1
  Switch3/1 -> aile/1
  aile_up/1 -> Switch3/3

== system rc_node/Manual Control/Radio Control Inputs/Subsystem ==
  In1 : Inport
  In2 : Inport  Port=2
  If Action Subsystem : Subsystem  TreatAsAtomicUnit=on
  If Action Subsystem1 : Subsystem  TreatAsAtomicUnit=on
  If1 : If  IfExpression=u1 == 0
  Merge : Merge
  Merge1 : Merge
  Out1 : Outport
  Out2 : Outport  Port=2
  wires:
  In1/1 -> If1/1, If Action Subsystem1/1(input)
  If1/1 -> If Action Subsystem/Action
  If1/2 -> If Action Subsystem1/Action
  If Action Subsystem1/1(Out1) -> Merge/2
  If Action Subsystem/1(Out1) -> Merge/1
  Merge/1 -> Out1/1
  In2/1 -> If Action Subsystem1/2(range)
  If Action Subsystem/2(Out2) -> Merge1/1
  If Action Subsystem1/2(Out2) -> Merge1/2
  Merge1/1 -> Out2/1

== system rc_node/Manual Control/Radio Control Inputs/Subsystem1 ==
  In1 : Inport
  In2 : Inport  Port=2
  If Action Subsystem2 : Subsystem  TreatAsAtomicUnit=on
  If Action Subsystem3 : Subsystem  TreatAsAtomicUnit=on
  If2 : If  IfExpression=u1 == 0
  Merge1 : Merge
  Merge2 : Merge
  Out1 : Outport
  Out2 : Outport  Port=2
  wires:
  In1/1 -> If Action Subsystem3/1(input), If2/1
  If2/1 -> If Action Subsystem2/Action
  If2/2 -> If Action Subsystem3/Action
  If Action Subsystem3/1(Out1) -> Merge1/2
  If Action Subsystem2/1(Out1) -> Merge1/1
  Merge1/1 -> Out1/1
  In2/1 -> If Action Subsystem3/2(range)
  If Action Subsystem2/2(Out2) -> Merge2/1
  Merge2/1 -> Out2/1
  If Action Subsystem3/2(Out2) -> Merge2/2

== system rc_node/Manual Control/Radio Control Inputs/Trigger rudder calibration ==
  in : Inport
  discon : Inport  Port=2
  mode : Inport  Port=3
  calState : Inport  Port=4
  Compare To Constant1 : simulink/Logic and Bit Operations/Compare To Constant  relop===  const=0  OutDataTypeStr=boolean
  Compute Calibration State : MATLAB Function  TreatAsAtomicUnit=on
  Detect Change1 : simulink/Logic and Bit Operations/Detect Change  vinit=0  InputProcessing=Inherited  OutDataTypeStr=boolean
  ECAN1 TX : Subsystem
  Logical Operator : Logic  AllPortsSameDT=off  OutDataTypeStr=boolean
  wires:
  Logical Operator/1 -> Compute Calibration State/1(trigger)
  Detect Change1/1 -> Logical Operator/1
  Compare To Constant1/1 -> Logical Operator/2
  mode/1 -> Compute Calibration State/2(mode)
  in/1 -> Detect Change1/1
  discon/1 -> Compare To Constant1/1
  Compute Calibration State/1(out) -> ECAN1 TX/Trigger
  calState/1 -> Compute Calibration State/3(calState)

== system rc_node/Manual Control/State outputs/If Action Subsystem1 ==
  Pulse : Inport
  Action Port : ActionPort  ActionType=then
  LED1 : Outport  InitialOutput=false
  wires:
  Pulse/1 -> LED1/1

== system rc_node/Manual Control/State outputs/If Action Subsystem2 ==
  Pulse : Inport
  Action Port : ActionPort  ActionType=elseif
  LED1 : Outport  InitialOutput=false
  wires:
  Pulse/1 -> LED1/1

== system rc_node/Manual Control/State outputs/If Action Subsystem3 ==
  Pulse : Inport
  Action Port : ActionPort  ActionType=elseif
  LED : Outport  InitialOutput=false
  wires:
  Pulse/1 -> LED/1

== system rc_node/Manual Control/State outputs/If Action Subsystem4 ==
  Action Port : ActionPort  ActionType=elseif
  Constant1 : Constant  Value=true  OutDataTypeStr=Inherit: Inherit via back propagation
  LED : Outport  InitialOutput=false
  wires:
  Constant1/1 -> LED/1
